simulink model "pid22"  (R2014a)
settings: Solver=ode23  StartTime=0.0  StopTime=20  RelTol=1e-3
settings Model: Creator=72395  LastModifiedBy=72395

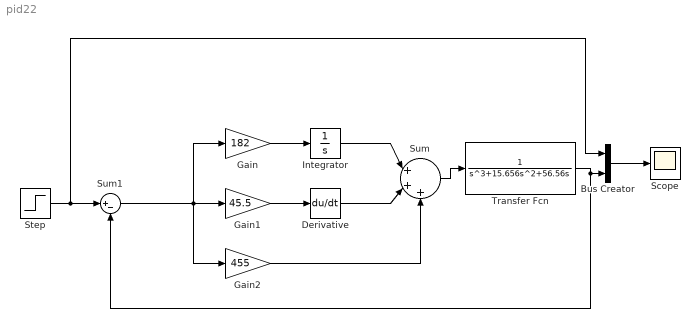
== system pid22 ==
  Bus Creator : BusCreator  Inputs=2
  Derivative : Derivative  CoefficientInTFapproximation=0
  Gain : Gain  Gain=182
  Gain1 : Gain  Gain=45.5
  Gain2 : Gain  Gain=455
  Integrator : Integrator
  Scope : Scope
      settings: TimeRange=20  YMin=0  YMax=2
  Step : Step  SampleTime=0
  Sum : Sum  Inputs=|+++
  Sum1 : Sum  Inputs=|+-
  Transfer Fcn : TransferFcn  Denominator=[1 15.656 56.56 0]
  wires:
  Sum1/1 -> Gain/1, Gain2/1, Gain1/1
  Gain/1 -> Integrator/1
  Gain1/1 -> Derivative/1
  Gain2/1 -> Sum/3
  Derivative/1 -> Sum/2
  Integrator/1 -> Sum/1
  Sum/1 -> Transfer Fcn/1
  Step/1 -> Bus Creator/1, Sum1/1
  Bus Creator/1 -> Scope/1
  Transfer Fcn/1 -> Sum1/2, Bus Creator/2
